simulink model "sampleModel1459"  (R2023a)
settings: Solver=VariableStepAuto  StartTime=0.0  StopTime=10.0  RelTol=1e-3
libraries: hdlsllib x5, simulink x2
settings Model: Creator=user1  LastModifiedBy=user1

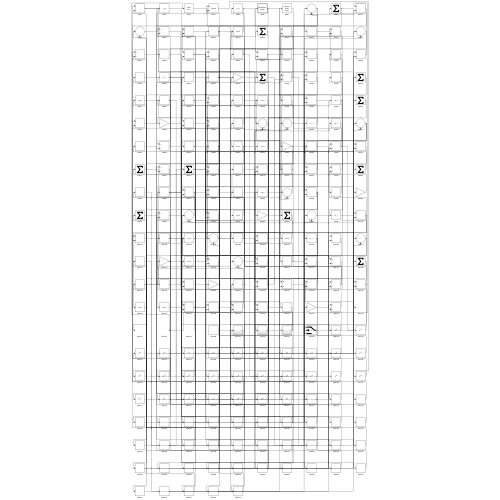
[thumbnail: Simulink's stored preview of the top-level diagram]
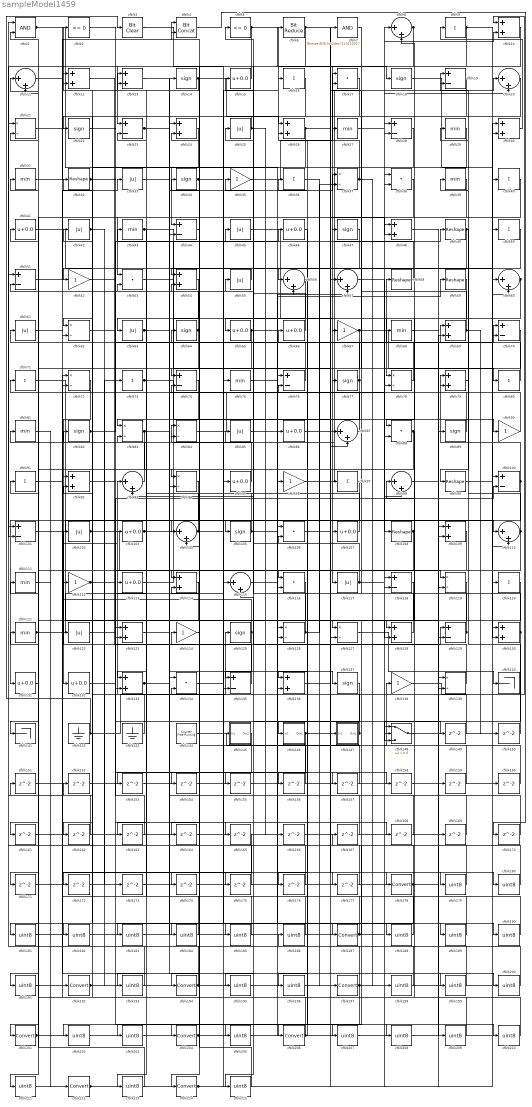
== system sampleModel1459 ==
  cfblk1 : Logic  AllPortsSameDT=off  OutDataTypeStr=boolean
  cfblk{10,12..13,24,26,30,48,54,69,79,92,109,114,123,128,130,133,136} (18 alike) : Sum
  cfblk{19,23,28,44,51,70,74,76,100..101,118,129,135} (13 alike) : Sum  Inputs=+-
  cfblk{25,33,42,45,55,61,63,85,102,117,122} (11 alike) : Abs  SaturateOnIntegerOverflow=off
  cfblk{15,41,46,65..66,86,95,103,107,113,131..132} (12 alike) : Bias  Bias=0.0  SaturateOnIntegerOverflow=off
  cfblk{8,11,20,56..57,60,87,93,98,104,110,115} (12 alike) : Sum  Inputs=|++
  cfblk{14,18,22,34,47,64,77,82,89,105,125,137} (12 alike) : Signum
  cfblk{17,38,53,88,106,116,134} (7 alike) : DotProduct  OutDataTypeStr=Inherit: Inherit via internal rule
  cfblk{32,49,58..59,99,108} (6 alike) : Reshape
  cfblk{27,29,31,39,43,68,75,81,111,121} (10 alike) : MinMax
  cfblk{35,52,67,90,96,112,124,138} (8 alike) : Gain
  cfblk{21,37,62,72,78,83..84,94,119,126..127,139} (12 alike) : Product  Inputs=*/  RndMeth=Zero  SaturateOnIntegerOverflow=on
  cfblk{9,16,36,40,50,71,73,80,91,97,120} (11 alike) : Sum  Inputs=+
  cfblk140 : Terminator
  cfblk141 : Terminator
  cfblk142 : Ground
  cfblk143 : Ground
  cfblk144 : hdlsllib/Sources/Counter Free-Running  NumBits=16  tsamp=-1
  cfblk145 : Subsystem
      settings: LibrarySourceBlock=|
      | hdlsllib/Ports &
      | Subsystems/Subsystem
  cfblk146 : Subsystem
      settings: LibrarySourceBlock=|
      | hdlsllib/Ports &
      | Subsystems/Subsystem
  cfblk147 : Subsystem
      settings: LibrarySourceBlock=|
      | hdlsllib/Ports &
      | Subsystems/Subsystem
  cfblk148 : Switch  SaturateOnIntegerOverflow=off  InputSameDT=off
  cfblk{149..177} (29 alike) : Delay  SampleTime=1
  cfblk{178,187,192,194,197,201,204,206,212,214} (10 alike) : DataTypeConversion  SaturateOnIntegerOverflow=off  RndMeth=Floor
  cfblk{179..186,188..191,193,195..196,198..200,202..203,205,207..211,213,215} (28 alike) : DataTypeConversion  OutDataTypeStr=uint8  SaturateOnIntegerOverflow=off  RndMeth=Floor
  cfblk2 : hdlsllib/Logic and Bit Operations/Compare To Zero  relop=<=  OutDataTypeStr=boolean
  cfblk3 : simulink/Logic and Bit Operations/Bit Clear  iBit=0
      settings: LibrarySourceBlock=|
      | hdlsllib/Logic and Bit
      | Operations/Bit Clear
  cfblk4 : hdlsllib/Logic and Bit Operations/Bit Concat  numInputs=2
  cfblk5 : hdlsllib/Logic and Bit Operations/Compare To Zero  relop=<=  OutDataTypeStr=boolean
  cfblk6 : hdlsllib/Logic and Bit Operations/Bit Reduce  mode=AND
  cfblk7 : simulink/Logic and Bit Operations/Bitwise Operator  logicop=AND  UseBitMask=on  BitMask=bin2dec('11011001')  BitMaskRealWorld=Stored Integer
      settings: LibrarySourceBlock=|
      | hdlsllib/Logic and Bit
      | Operations/Bitwise
      | Operator
  wires:
  cfblk103/1 -> cfblk45/1, cfblk13/2
  cfblk126/1 -> cfblk84/1, cfblk37/2
  cfblk20/1 -> cfblk105/1
  cfblk15/1 -> cfblk23/1
  cfblk12/1 -> cfblk129/1
  cfblk106/1 -> cfblk178/1
  cfblk72/1 -> cfblk132/1
  cfblk42/1 -> cfblk172/1, cfblk173/1
  cfblk95/1 -> cfblk11/1
  cfblk78/1 -> cfblk58/1
  cfblk66/1 -> cfblk25/1
  cfblk120/1 -> cfblk204/1
  cfblk26/1 -> cfblk62/1, cfblk48/2
  cfblk37/1 -> cfblk6/1, cfblk198/1
  cfblk146/1(Out1) -> cfblk70/2, cfblk155/1
  cfblk8/1 -> cfblk117/1, cfblk101/2
  cfblk96/1 -> cfblk49/1
  cfblk76/1 -> cfblk35/1
  cfblk5/1 -> cfblk18/1, cfblk164/1
  cfblk101/1 -> cfblk107/1
  cfblk81/1 -> cfblk192/1
  cfblk14/1 -> cfblk26/1, cfblk12/2
  cfblk127/1 -> cfblk140/1
  cfblk21/1 -> cfblk96/1
  cfblk134/1 -> cfblk187/1
  cfblk128/1 -> cfblk17/1
  cfblk79/1 -> cfblk39/1
  cfblk64/1 -> cfblk42/1, cfblk72/2, cfblk171/1
  cfblk86/1 -> cfblk7/1
  cfblk108/1 -> cfblk191/1, cfblk203/1
  cfblk3/1 -> cfblk95/1
  cfblk30/1 -> cfblk9/1
  cfblk1/1 -> cfblk126/1, cfblk180/1
  cfblk77/1 -> cfblk4/1, cfblk94/2
  cfblk109/1 -> cfblk206/1
  cfblk89/1 -> cfblk15/1
  cfblk97/1 -> cfblk131/1
  cfblk16/1 -> cfblk52/1
  cfblk113/1 -> cfblk20/1
  cfblk144/1 -> cfblk138/1
  cfblk53/1 -> cfblk67/1
  cfblk88/1 -> cfblk128/1, cfblk141/1, cfblk153/1
  cfblk143/1 -> cfblk93/1
  cfblk142/1 -> cfblk3/1, cfblk125/1
  cfblk29/1 -> cfblk44/1
  cfblk74/1 -> cfblk83/1
  cfblk117/1 -> cfblk55/1, cfblk20/2
  cfblk44/1 -> cfblk104/1
  cfblk18/1 -> cfblk130/1
  cfblk83/1 -> cfblk69/1, cfblk133/2
  cfblk6/1 -> cfblk62/2, cfblk87/2
  cfblk71/1 -> cfblk127/1
  cfblk139/1 -> cfblk115/2
  cfblk90/1 -> cfblk29/1
  cfblk23/1 -> cfblk56/1, cfblk200/1
  cfblk112/1 -> cfblk162/1, cfblk210/1
  cfblk51/1 -> cfblk33/1
  cfblk100/1 -> cfblk79/1, cfblk135/2, cfblk161/1
  cfblk58/1 -> cfblk5/1
  cfblk124/1 -> cfblk214/1
  cfblk35/1 -> cfblk17/2
  cfblk59/1 -> cfblk78/1
  cfblk25/1 -> cfblk22/1, cfblk166/1
  cfblk87/1 -> cfblk11/2
  cfblk130/1 -> cfblk93/2, cfblk148/2
  cfblk57/1 -> cfblk108/1
  cfblk41/1 -> cfblk60/2
  cfblk125/1 -> cfblk102/1, cfblk135/1
  cfblk19/1 -> cfblk74/1
  cfblk107/1 -> cfblk61/1
  cfblk11/1 -> cfblk2/1
  cfblk111/1 -> cfblk212/1
  cfblk131/1 -> cfblk31/1
  cfblk104/1 -> cfblk71/1, cfblk110/1, cfblk148/3
  cfblk123/1 -> cfblk37/1
  cfblk43/1 -> cfblk127/2, cfblk63/1
  cfblk9/1 -> cfblk130/2, cfblk27/1
  cfblk49/1 -> cfblk99/1, cfblk196/1
  cfblk45/1 -> cfblk97/1
  cfblk133/1 -> cfblk137/1, cfblk70/1
  cfblk60/1 -> cfblk88/1, cfblk146/1(In1), cfblk88/2
  cfblk39/1 -> cfblk53/1
  cfblk136/1 -> cfblk19/1
  cfblk135/1 -> cfblk112/1
  cfblk28/1 -> cfblk194/1
  cfblk63/1 -> cfblk23/2, cfblk128/2
  cfblk138/1 -> cfblk10/1
  cfblk80/1 -> cfblk12/1
  cfblk82/1 -> cfblk46/1, cfblk68/1, cfblk177/1
  cfblk67/1 -> cfblk80/1, cfblk133/1
  cfblk36/1 -> cfblk197/1
  cfblk102/1 -> cfblk119/1, cfblk119/2
  cfblk73/1 -> cfblk139/2, cfblk76/2
  cfblk129/1 -> cfblk51/2, cfblk85/1
  cfblk48/1 -> cfblk90/1
  cfblk121/1 -> cfblk16/1, cfblk103/1
  cfblk68/1 -> cfblk89/1
  cfblk40/1 -> cfblk47/1
  cfblk148/1 -> cfblk100/1
  cfblk110/1 -> cfblk114/1, cfblk122/1, cfblk79/2
  cfblk122/1 -> cfblk100/2
  cfblk147/1(Out1) -> cfblk53/2, cfblk82/1
  cfblk46/1 -> cfblk136/1
  cfblk105/1 -> cfblk136/2, cfblk13/1
  cfblk32/1 -> cfblk116/1, cfblk158/1
  cfblk93/1 -> cfblk41/1
  cfblk13/1 -> cfblk116/2
  cfblk10/1 -> cfblk65/1
  cfblk34/1 -> cfblk129/2, cfblk168/1
  cfblk99/1 -> cfblk50/1
  cfblk118/1 -> cfblk201/1
  cfblk69/1 -> cfblk43/1, cfblk150/1
  cfblk24/1 -> cfblk123/2
  cfblk55/1 -> cfblk54/1
  cfblk65/1 -> cfblk94/1, cfblk59/1
  cfblk7/1 -> cfblk77/1
  cfblk31/1 -> cfblk4/2
  cfblk27/1 -> cfblk10/2
  cfblk84/1 -> cfblk8/1
  cfblk115/1 -> cfblk57/2
  cfblk62/1 -> cfblk149/1
  cfblk149/1 -> cfblk54/2
  cfblk150/1 -> cfblk19/2
  cfblk151/1 -> cfblk126/2
  cfblk153/1 -> cfblk48/1
  cfblk17/1 -> cfblk154/1
  cfblk154/1 -> cfblk30/1
  cfblk155/1 -> cfblk60/1
  cfblk70/1 -> cfblk156/1
  cfblk156/1 -> cfblk84/2
  cfblk33/1 -> cfblk157/1
  cfblk157/1 -> cfblk114/2
  cfblk158/1 -> cfblk110/2
  cfblk159/1 -> cfblk148/1
  cfblk160/1 -> cfblk8/2
  cfblk161/1 -> cfblk69/2
  cfblk162/1 -> cfblk1/1
  cfblk94/1 -> cfblk163/1
  cfblk163/1 -> cfblk123/1
  cfblk164/1 -> cfblk78/2
  cfblk132/1 -> cfblk165/1
  cfblk166/1 -> cfblk87/1
  cfblk167/1 -> cfblk74/2
  cfblk168/1 -> cfblk26/2
  cfblk169/1 -> cfblk24/1
  cfblk4/1 -> cfblk170/1
  cfblk170/1 -> cfblk104/2
  cfblk171/1 -> cfblk139/1
  cfblk172/1 -> cfblk115/1
  cfblk173/1 -> cfblk44/2
  cfblk52/1 -> cfblk174/1
  cfblk174/1 -> cfblk57/1
  cfblk61/1 -> cfblk175/1
  cfblk175/1 -> cfblk21/1
  cfblk47/1 -> cfblk176/1
  cfblk176/1 -> cfblk83/2
  cfblk177/1 -> cfblk1/2
  cfblk178/1 -> cfblk51/1, cfblk211/1
  cfblk85/1 -> cfblk179/1
  cfblk179/1 -> cfblk106/1
  cfblk180/1 -> cfblk106/2
  cfblk38/1 -> cfblk181/1
  cfblk181/1 -> cfblk14/1
  cfblk165/1 -> cfblk182/1
  cfblk182/1 -> cfblk38/1
  cfblk54/1 -> cfblk183/1
  cfblk183/1 -> cfblk38/2
  cfblk92/1 -> cfblk184/1
  cfblk184/1 -> cfblk152/1
  cfblk116/1 -> cfblk185/1
  cfblk185/1 -> cfblk92/1
  cfblk186/1 -> cfblk92/2
  cfblk187/1 -> cfblk167/1, cfblk34/1, cfblk66/1
  cfblk2/1 -> cfblk188/1
  cfblk188/1 -> cfblk134/1
  cfblk152/1 -> cfblk189/1
  cfblk189/1 -> cfblk134/2
  cfblk75/1 -> cfblk190/1
  cfblk190/1 -> cfblk113/1
  cfblk191/1 -> cfblk75/1
  cfblk192/1 -> cfblk76/1, cfblk73/1
  cfblk145/1(Out1) -> cfblk193/1
  cfblk193/1 -> cfblk81/1
  cfblk194/1 -> cfblk101/1, cfblk121/1
  cfblk50/1 -> cfblk195/1
  cfblk195/1 -> cfblk28/1
  cfblk196/1 -> cfblk28/2
  cfblk197/1 -> cfblk40/1, cfblk21/2, cfblk202/1
  cfblk198/1 -> cfblk36/1
  cfblk91/1 -> cfblk199/1
  cfblk199/1 -> cfblk24/2
  cfblk200/1 -> cfblk91/1
  cfblk201/1 -> cfblk169/1, cfblk56/2
  cfblk202/1 -> cfblk118/1
  cfblk203/1 -> cfblk118/2
  cfblk204/1 -> cfblk64/1, cfblk86/1
  cfblk56/1 -> cfblk205/1
  cfblk205/1 -> cfblk120/1
  cfblk206/1 -> cfblk186/1, cfblk151/1, cfblk72/1, cfblk30/2
  cfblk119/1 -> cfblk207/1
  cfblk207/1 -> cfblk109/1
  cfblk22/1 -> cfblk208/1
  cfblk208/1 -> cfblk109/2
  cfblk98/1 -> cfblk209/1
  cfblk209/1 -> cfblk32/1
  cfblk210/1 -> cfblk98/1
  cfblk211/1 -> cfblk98/2
  cfblk212/1 -> cfblk147/1(In1), cfblk145/1(In1)
  cfblk114/1 -> cfblk213/1
  cfblk213/1 -> cfblk111/1
  cfblk214/1 -> cfblk160/1, cfblk159/1
  cfblk137/1 -> cfblk215/1
  cfblk215/1 -> cfblk124/1

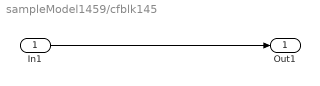
== system sampleModel1459/cfblk145 ==
  In1 : Inport
  Out1 : Outport
  wires:
  In1/1 -> Out1/1

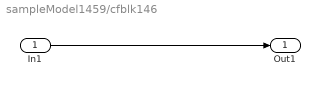
== system sampleModel1459/cfblk146 ==
  In1 : Inport
  Out1 : Outport
  wires:
  In1/1 -> Out1/1

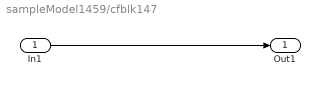
== system sampleModel1459/cfblk147 ==
  In1 : Inport
  Out1 : Outport
  wires:
  In1/1 -> Out1/1
